simulink model "chaser_target_slosh"  (R2024a)
settings: Solver=VariableStepAuto  StartTime=0.0  StopTime=10.0  RelTol=1e-3
values from neighbouring files (symbols this model uses):
  dispslosh = 0.2    [main.m]
undefined symbols (not defined in the file or in its folder): chaser, InvDyn, KIN, reaction_wheels, slosh, solar_panel_big_reduced_FEM, solar_panel_target_reduced_FEM, target, ureal, uss, wn_big, wn_target
libraries: RCTblocks x54, SDTlibV1 x44
(part 2 of 3)

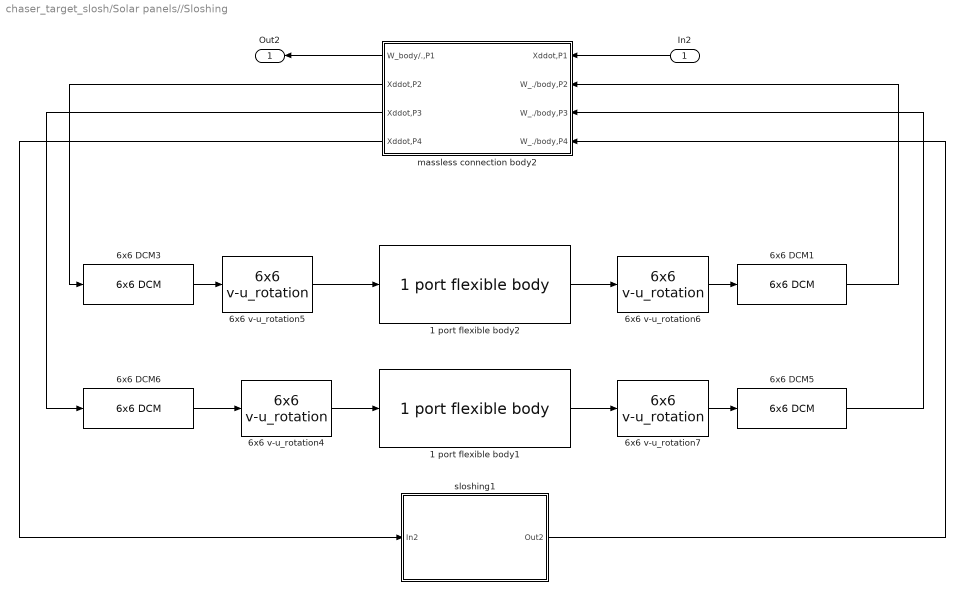
== system chaser_target_slosh/Solar panels//Sloshing ==
  In2 : Inport
  1 port flexible body1 : SDTlibV1/6 dof bodies/1 port flexible body  m=solar_panel_big_reduced_FEM.m  Ig=inertias_big  OG=r_PG_big  OP=[0;0;0]  n=6  xi=solar_panel_big_reduced_FEM.xi  w1=ureal('wnbig1',wn_big(1),'Percentage',20);  L11=solar_panel_big_reduced_FEM.L(1,1)  L12=solar_panel_big_reduced_FEM.L(1,2)  L13=solar_panel_big_reduced_FEM.L(1,3)  L14=solar_panel_big_reduced_FEM.L(1,4)  L15=solar_panel_big_reduced_FEM.L(1,5)  L16=solar_panel_big_reduced_FEM.L(1,6)  w2=wn_big(2)  L21=solar_panel_big_reduced_FEM.L(2,1)  L22=solar_panel_big_reduced_FEM.L(2,2)  L23=solar_panel_big_reduced_FEM.L(2,3)  L24=solar_panel_big_reduced_FEM.L(2,4)  L25=solar_panel_big_reduced_FEM.L(2,5)  L26=solar_panel_big_reduced_FEM.L(2,6)  w3=wn_big(3)  L31=solar_panel_big_reduced_FEM.L(3,1)  L32=solar_panel_big_reduced_FEM.L(3,2)  L33=solar_panel_big_reduced_FEM.L(3,3)  L34=solar_panel_big_reduced_FEM.L(3,4)  L35=solar_panel_big_reduced_FEM.L(3,5)  L36=solar_panel_big_reduced_FEM.L(3,6)  w4=wn_big(4)  L41=solar_panel_big_reduced_FEM.L(4,1)  L42=solar_panel_big_reduced_FEM.L(4,2)  L43=solar_panel_big_reduced_FEM.L(4,3)  L44=solar_panel_big_reduced_FEM.L(4,4)  L45=solar_panel_big_reduced_FEM.L(4,5)  L46=solar_panel_big_reduced_FEM.L(4,6)  w5=wn_big(5)  L51=solar_panel_big_reduced_FEM.L(5,1)  L52=solar_panel_big_reduced_FEM.L(5,2)  L53=solar_panel_big_reduced_FEM.L(5,3)  L54=solar_panel_big_reduced_FEM.L(5,4)  L55=solar_panel_big_reduced_FEM.L(5,5)  L56=solar_panel_big_reduced_FEM.L(5,6)  w6=wn_big(6)  L61=solar_panel_big_reduced_FEM.L(6,1)  L62=solar_panel_big_reduced_FEM.L(6,2)  L63=solar_panel_big_reduced_FEM.L(6,3)  L64=solar_panel_big_reduced_FEM.L(6,4)  L65=solar_panel_big_reduced_FEM.L(6,5)  L66=solar_panel_big_reduced_FEM.L(6,6)  w7=0  L71=0  L72=0  L73=0  L74=0  L75=0  L76=0  w8=0  L81=0  L82=0  L83=0  L84=0  L85=0  L86=0  w9=0  L91=0  L92=0  L93=0  L94=0  L95=0  L96=0  w10=0  L101=0  L102=0  L103=0  L104=0  L105=0  L106=0
      settings: SourceProductName=SDTlib
  1 port flexible body2 : SDTlibV1/6 dof bodies/1 port flexible body  m=solar_panel_big_reduced_FEM.m  Ig=inertias_big  OG=r_PG_big  OP=[0;0;0]  n=6  xi=solar_panel_big_reduced_FEM.xi  w1=ureal('wnbig1',wn_big(1),'Percentage',20);  L11=solar_panel_big_reduced_FEM.L(1,1)  L12=solar_panel_big_reduced_FEM.L(1,2)  L13=solar_panel_big_reduced_FEM.L(1,3)  L14=solar_panel_big_reduced_FEM.L(1,4)  L15=solar_panel_big_reduced_FEM.L(1,5)  L16=solar_panel_big_reduced_FEM.L(1,6)  w2=wn_big(2)  L21=solar_panel_big_reduced_FEM.L(2,1)  L22=solar_panel_big_reduced_FEM.L(2,2)  L23=solar_panel_big_reduced_FEM.L(2,3)  L24=solar_panel_big_reduced_FEM.L(2,4)  L25=solar_panel_big_reduced_FEM.L(2,5)  L26=solar_panel_big_reduced_FEM.L(2,6)  w3=wn_big(3)  L31=solar_panel_big_reduced_FEM.L(3,1)  L32=solar_panel_big_reduced_FEM.L(3,2)  L33=solar_panel_big_reduced_FEM.L(3,3)  L34=solar_panel_big_reduced_FEM.L(3,4)  L35=solar_panel_big_reduced_FEM.L(3,5)  L36=solar_panel_big_reduced_FEM.L(3,6)  w4=wn_big(4)  L41=solar_panel_big_reduced_FEM.L(4,1)  L42=solar_panel_big_reduced_FEM.L(4,2)  L43=solar_panel_big_reduced_FEM.L(4,3)  L44=solar_panel_big_reduced_FEM.L(4,4)  L45=solar_panel_big_reduced_FEM.L(4,5)  L46=solar_panel_big_reduced_FEM.L(4,6)  w5=wn_big(5)  L51=solar_panel_big_reduced_FEM.L(5,1)  L52=solar_panel_big_reduced_FEM.L(5,2)  L53=solar_panel_big_reduced_FEM.L(5,3)  L54=solar_panel_big_reduced_FEM.L(5,4)  L55=solar_panel_big_reduced_FEM.L(5,5)  L56=solar_panel_big_reduced_FEM.L(5,6)  w6=wn_big(6)  L61=solar_panel_big_reduced_FEM.L(6,1)  L62=solar_panel_big_reduced_FEM.L(6,2)  L63=solar_panel_big_reduced_FEM.L(6,3)  L64=solar_panel_big_reduced_FEM.L(6,4)  L65=solar_panel_big_reduced_FEM.L(6,5)  L66=solar_panel_big_reduced_FEM.L(6,6)  w7=0  L71=0  L72=0  L73=0  L74=0  L75=0  L76=0  w8=0  L81=0  L82=0  L83=0  L84=0  L85=0  L86=0  w9=0  L91=0  L92=0  L93=0  L94=0  L95=0  L96=0  w10=0  L101=0  L102=0  L103=0  L104=0  L105=0  L106=0
      settings: SourceProductName=SDTlib
  6x6 DCM1 : SDTlibV1/3//6 dof DCM/6x6 DCM  rot=chaser.solarpanel.R(:,:,1)  transp=off
      settings: SourceProductName=SDTlib
  6x6 DCM3 : SDTlibV1/3//6 dof DCM/6x6 DCM  rot=chaser.solarpanel.R(:,:,1)  transp=on
      settings: SourceProductName=SDTlib
  6x6 DCM5 : SDTlibV1/3//6 dof DCM/6x6 DCM  rot=chaser.solarpanel.R(:,:,2)  transp=off
      settings: SourceProductName=SDTlib
  6x6 DCM6 : SDTlibV1/3//6 dof DCM/6x6 DCM  rot=chaser.solarpanel.R(:,:,2)  transp=on
      settings: SourceProductName=SDTlib
  6x6 v-u_rotation4 : SDTlibV1/3//6 dof DCM/6x6 v-u_rotation  ra=[0;1;0]  theta=ureal('theta8',0,'Range',[-pi pi])  transp=on
      settings: SourceProductName=SDTlib
  6x6 v-u_rotation5 : SDTlibV1/3//6 dof DCM/6x6 v-u_rotation  ra=[0;1;0]  theta=ureal('theta7',0,'Range',[-pi pi])  transp=on
      settings: SourceProductName=SDTlib
  6x6 v-u_rotation6 : SDTlibV1/3//6 dof DCM/6x6 v-u_rotation  ra=[0;1;0]  theta=ureal('theta7',0,'Range',[-pi pi])  transp=off
      settings: SourceProductName=SDTlib
  6x6 v-u_rotation7 : SDTlibV1/3//6 dof DCM/6x6 v-u_rotation  ra=[0;1;0]  theta=ureal('theta8',0,'Range',[-pi pi])  transp=off
      settings: SourceProductName=SDTlib
  massless connection body2 : Subsystem  mask(Massless multi_port (6nx6n)){n=4, numinv=1, OP1=[0;0;0], OP2=chaser.solarpanel.location(:,1)*0.9, OP3=chaser.solarpanel.location(:,2)*0.9, OP4=[0;0;0], OP5=chaser.GNC.control.reaction_wheels.positions(:,4), OP6=[0;0;0], OP7=[0;0;0]}
      mask prompts: n "Number of ports"; numinv "Port (point) Pj: j="; OP1 "OP1 (3x1 vector, m)"; OP2 "OP2 (3x1 vector, m)"; OP3 "OP3 (3x1 vector, m)"; OP4 "OP4 (3x1 vector, m)"; OP5 "OP5 (3x1 vector,m)"; OP6 "OP6 (3x1 vector,m)"; OP7 "OP7 (3x1 vector,m)"
      mask help:
      | Massless body to transport wrenches and acceleration twists:
      | 6nx6n gain from:
      |  * the acceleration twist at one point Pj; i.e. the parent port,
      |  * the wrenches applied to this massless body at the n-1 points Pi (i=1,..n, except j); i.e. the child ports
      | to:
      |  * the wrench applied at point Pj by this massless body,
      |  * the accelaretion twists at the other n-1  points Pi (i=1,..n, except j).
      |
      | 0: the reference point
      | Pi (i=1:n): the n given connection points or ports (1<n<8).
      |
      | All parameters are expressed in the body frame.
      | Each parameter can be an uncertain parameter declared with "ureal"
      mask init:
      | MasslessConnectionBody
      mask Help: web('DocMassLessBody.html')
      mask TypeOptions n: 2 | 3 | 4 | 5 | 6 | 7
      mask TypeOptions numinv: 1 | 2 | 3 | 4 | 5 | 6 | 7
      mask DialogControl ParameterGroupVar Prompt: Main parameters
      mask DialogControl port1 Prompt: Port #1
      mask DialogControl port2 Prompt: #2
      mask DialogControl port3 Prompt: #3
      mask DialogControl port4 Prompt: #4
      mask DialogControl port5 Prompt: #5
      mask DialogControl port6 Prompt: #6
      mask DialogControl port7 Prompt: #7
      mask Display:
      | disp('Massless\n connection body\n (6nx6n)')
      | for ii=1:n+1
      |     if numinv==ii,
      |         port_label('output',ii,['W_body/.,P',num2str(ii)])
      |         port_label('input', ii,['Xddot,P',num2str(ii)])
      |     else
      |         port_label('input', ii,['W_./body,P',num2str(ii)])
      |         port_label('output',ii,['Xddot,P',num2str(ii)])
      |     end
      | end
  sloshing1 : Subsystem
  Out2 : Outport
  wires:
  massless connection body2/1(W_body/.,P1) -> Out2/1
  In2/1 -> massless connection body2/1(Xddot,P1)
  1 port flexible body2/1 -> 6x6 v-u_rotation6/1
  6x6 v-u_rotation5/1 -> 1 port flexible body2/1
  6x6 v-u_rotation6/1 -> 6x6 DCM1/1
  1 port flexible body1/1 -> 6x6 v-u_rotation7/1
  massless connection body2/2(Xddot,P2) -> 6x6 DCM3/1
  6x6 DCM1/1 -> massless connection body2/2(W_./body,P2)
  6x6 DCM3/1 -> 6x6 v-u_rotation5/1
  6x6 v-u_rotation7/1 -> 6x6 DCM5/1
  6x6 DCM5/1 -> massless connection body2/3(W_./body,P3)
  massless connection body2/3(Xddot,P3) -> 6x6 DCM6/1
  6x6 DCM6/1 -> 6x6 v-u_rotation4/1
  6x6 v-u_rotation4/1 -> 1 port flexible body1/1
  massless connection body2/4(Xddot,P4) -> sloshing1/1(In2)
  sloshing1/1(Out2) -> massless connection body2/4(W_./body,P4)

== system chaser_target_slosh/Reaction Wheels 0 vel1/RW1 ==
  Xddot : Inport  PortDimensions=6
  Demux : Demux  Outputs=[3 3]
  Gain1 : Gain  Gain=pass'  Multiplication=Matrix(K*u) (u vector)
  Gain2 : Gain  Gain=pass  Multiplication=Matrix(K*u) (u vector)
  Gain3 : Gain  Gain=m*eye(3)  Multiplication=Matrix(K*u) (u vector)
  Gain4 : Gain  Gain=diag([Ir Ir Iw])  Multiplication=Matrix(K*u) (u vector)
  Gain8 : Gain  Gain=-Tau_GP'  Multiplication=Matrix(K*u) (u vector)
  Gain9 : Gain  Gain=Tau_GP  Multiplication=Matrix(K*u) (u vector)
  Mux : Mux  Inputs=[3 3]
  W_body/. : Outport  VectorParamsAs1DForOutWhenUnconnected=off
  wires:
  Gain3/1 -> Mux/1
  Gain2/1 -> Mux/2
  Demux/1 -> Gain3/1
  Demux/2 -> Gain1/1
  Gain1/1 -> Gain4/1
  Gain4/1 -> Gain2/1
  Gain8/1 -> W_body/./1
  Mux/1 -> Gain8/1
  Gain9/1 -> Demux/1
  Xddot/1 -> Gain9/1

== system chaser_target_slosh/Reaction Wheels 0 vel1/RW2 ==
  Xddot : Inport  PortDimensions=6
  Demux : Demux  Outputs=[3 3]
  Gain1 : Gain  Gain=pass'  Multiplication=Matrix(K*u) (u vector)
  Gain2 : Gain  Gain=pass  Multiplication=Matrix(K*u) (u vector)
  Gain3 : Gain  Gain=m*eye(3)  Multiplication=Matrix(K*u) (u vector)
  Gain4 : Gain  Gain=diag([Ir Ir Iw])  Multiplication=Matrix(K*u) (u vector)
  Gain8 : Gain  Gain=-Tau_GP'  Multiplication=Matrix(K*u) (u vector)
  Gain9 : Gain  Gain=Tau_GP  Multiplication=Matrix(K*u) (u vector)
  Mux : Mux  Inputs=[3 3]
  W_body/. : Outport  VectorParamsAs1DForOutWhenUnconnected=off
  wires:
  Gain3/1 -> Mux/1
  Gain2/1 -> Mux/2
  Demux/1 -> Gain3/1
  Demux/2 -> Gain1/1
  Gain1/1 -> Gain4/1
  Gain4/1 -> Gain2/1
  Gain8/1 -> W_body/./1
  Mux/1 -> Gain8/1
  Gain9/1 -> Demux/1
  Xddot/1 -> Gain9/1

== system chaser_target_slosh/Reaction Wheels 0 vel1/RW3 ==
  Xddot : Inport  PortDimensions=6
  Demux : Demux  Outputs=[3 3]
  Gain1 : Gain  Gain=pass'  Multiplication=Matrix(K*u) (u vector)
  Gain2 : Gain  Gain=pass  Multiplication=Matrix(K*u) (u vector)
  Gain3 : Gain  Gain=m*eye(3)  Multiplication=Matrix(K*u) (u vector)
  Gain4 : Gain  Gain=diag([Ir Ir Iw])  Multiplication=Matrix(K*u) (u vector)
  Gain8 : Gain  Gain=-Tau_GP'  Multiplication=Matrix(K*u) (u vector)
  Gain9 : Gain  Gain=Tau_GP  Multiplication=Matrix(K*u) (u vector)
  Mux : Mux  Inputs=[3 3]
  W_body/. : Outport  VectorParamsAs1DForOutWhenUnconnected=off
  wires:
  Gain3/1 -> Mux/1
  Gain2/1 -> Mux/2
  Demux/1 -> Gain3/1
  Demux/2 -> Gain1/1
  Gain1/1 -> Gain4/1
  Gain4/1 -> Gain2/1
  Gain8/1 -> W_body/./1
  Mux/1 -> Gain8/1
  Gain9/1 -> Demux/1
  Xddot/1 -> Gain9/1

== system chaser_target_slosh/Reaction Wheels 0 vel1/RW4 ==
  Xddot : Inport  PortDimensions=6
  Demux : Demux  Outputs=[3 3]
  Gain1 : Gain  Gain=pass'  Multiplication=Matrix(K*u) (u vector)
  Gain2 : Gain  Gain=pass  Multiplication=Matrix(K*u) (u vector)
  Gain3 : Gain  Gain=m*eye(3)  Multiplication=Matrix(K*u) (u vector)
  Gain4 : Gain  Gain=diag([Ir Ir Iw])  Multiplication=Matrix(K*u) (u vector)
  Gain8 : Gain  Gain=-Tau_GP'  Multiplication=Matrix(K*u) (u vector)
  Gain9 : Gain  Gain=Tau_GP  Multiplication=Matrix(K*u) (u vector)
  Mux : Mux  Inputs=[3 3]
  W_body/. : Outport  VectorParamsAs1DForOutWhenUnconnected=off
  wires:
  Gain3/1 -> Mux/1
  Gain2/1 -> Mux/2
  Demux/1 -> Gain3/1
  Demux/2 -> Gain1/1
  Gain1/1 -> Gain4/1
  Gain4/1 -> Gain2/1
  Gain8/1 -> W_body/./1
  Mux/1 -> Gain8/1
  Gain9/1 -> Demux/1
  Xddot/1 -> Gain9/1

== system chaser_target_slosh/Reaction Wheels 0 vel1/massless connection body1 ==
  Xddot,P1 : Inport  PortDimensions=6
  W_./body,P2 : Inport  Port=2  PortDimensions=6
  W_./body,P3 : Inport  Port=3  PortDimensions=6
  W_./body,P4 : Inport  Port=4  PortDimensions=6
  W_./body,P5 : Inport  Port=5  PortDimensions=6
  Demux : Demux  Outputs=[6 6 6 6 6]
  Gain : RCTblocks/Uncertain State Space  Tag=USS  USystem=uss(KIN)  UValue=[]  X0=[]  uX0=[]
  Mux : Mux  Inputs=[6 6 6 6 6]
  W_body/.,P1 : Outport
  Xddot,P2 : Outport  Port=2
  Xddot,P3 : Outport  Port=3
  Xddot,P4 : Outport  Port=4
  Xddot,P5 : Outport  Port=5
  wires:
  Mux/1 -> Gain/1
  Gain/1 -> Demux/1
  Xddot,P1/1 -> Mux/1
  Demux/1 -> W_body/.,P1/1
  W_./body,P2/1 -> Mux/2
  Demux/2 -> Xddot,P2/1
  W_./body,P3/1 -> Mux/3
  Demux/3 -> Xddot,P3/1
  W_./body,P4/1 -> Mux/4
  Demux/4 -> Xddot,P4/1
  W_./body,P5/1 -> Mux/5
  Demux/5 -> Xddot,P5/1

== system chaser_target_slosh/Robotic arm/Multi port rigid body1 ==
  Xddot,P1 : Inport  PortDimensions=6
  W_./body,P2 : Inport  Port=2  PortDimensions=6
  Demux : Demux  Outputs=[6 6]
  Gain : RCTblocks/Uncertain State Space  Tag=USS  USystem=uss(InvDyn)  UValue=[]  X0=[]  uX0=[]
  Mux : Mux  Inputs=[6 6]
  W_body/.,P1 : Outport
  Xddot,P2 : Outport  Port=2
  wires:
  Mux/1 -> Gain/1
  Gain/1 -> Demux/1
  Xddot,P1/1 -> Mux/1
  Demux/1 -> W_body/.,P1/1
  W_./body,P2/1 -> Mux/2
  Demux/2 -> Xddot,P2/1

== system chaser_target_slosh/Robotic arm/Multi port rigid body3 ==
  Xddot,P1 : Inport  PortDimensions=6
  W_./body,P2 : Inport  Port=2  PortDimensions=6
  Demux : Demux  Outputs=[6 6]
  Gain : RCTblocks/Uncertain State Space  Tag=USS  USystem=uss(InvDyn)  UValue=[]  X0=[]  uX0=[]
  Mux : Mux  Inputs=[6 6]
  W_body/.,P1 : Outport
  Xddot,P2 : Outport  Port=2
  wires:
  Mux/1 -> Gain/1
  Gain/1 -> Demux/1
  Xddot,P1/1 -> Mux/1
  Demux/1 -> W_body/.,P1/1
  W_./body,P2/1 -> Mux/2
  Demux/2 -> Xddot,P2/1

== system chaser_target_slosh/Robotic arm/Multi port rigid body4 ==
  Xddot,P1 : Inport  PortDimensions=6
  W_./body,P2 : Inport  Port=2  PortDimensions=6
  Demux : Demux  Outputs=[6 6]
  Gain : RCTblocks/Uncertain State Space  Tag=USS  USystem=uss(InvDyn)  UValue=[]  X0=[]  uX0=[]
  Mux : Mux  Inputs=[6 6]
  W_body/.,P1 : Outport
  Xddot,P2 : Outport  Port=2
  wires:
  Mux/1 -> Gain/1
  Gain/1 -> Demux/1
  Xddot,P1/1 -> Mux/1
  Demux/1 -> W_body/.,P1/1
  W_./body,P2/1 -> Mux/2
  Demux/2 -> Xddot,P2/1

== system chaser_target_slosh/Robotic arm/Multi port rigid body6 ==
  Xddot,P1 : Inport  PortDimensions=6
  W_./body,P2 : Inport  Port=2  PortDimensions=6
  Demux : Demux  Outputs=[6 6]
  Gain : RCTblocks/Uncertain State Space  Tag=USS  USystem=uss(InvDyn)  UValue=[]  X0=[]  uX0=[]
  Mux : Mux  Inputs=[6 6]
  W_body/.,P1 : Outport
  Xddot,P2 : Outport  Port=2
  wires:
  Mux/1 -> Gain/1
  Gain/1 -> Demux/1
  Xddot,P1/1 -> Mux/1
  Demux/1 -> W_body/.,P1/1
  W_./body,P2/1 -> Mux/2
  Demux/2 -> Xddot,P2/1

== system chaser_target_slosh/Robotic arm/Multi port rigid body7 ==
  Xddot,P1 : Inport  PortDimensions=6
  W_./body,P2 : Inport  Port=2  PortDimensions=6
  Demux : Demux  Outputs=[6 6]
  Gain : RCTblocks/Uncertain State Space  Tag=USS  USystem=uss(InvDyn)  UValue=[]  X0=[]  uX0=[]
  Mux : Mux  Inputs=[6 6]
  W_body/.,P1 : Outport
  Xddot,P2 : Outport  Port=2
  wires:
  Mux/1 -> Gain/1
  Gain/1 -> Demux/1
  Xddot,P1/1 -> Mux/1
  Demux/1 -> W_body/.,P1/1
  W_./body,P2/1 -> Mux/2
  Demux/2 -> Xddot,P2/1

== system chaser_target_slosh/Robotic arm/Multi port rigid body8 ==
  Xddot,P1 : Inport  PortDimensions=6
  W_./body,P2 : Inport  Port=2  PortDimensions=6
  Demux : Demux  Outputs=[6 6]
  Gain : RCTblocks/Uncertain State Space  Tag=USS  USystem=uss(InvDyn)  UValue=[]  X0=[]  uX0=[]
  Mux : Mux  Inputs=[6 6]
  W_body/.,P1 : Outport
  Xddot,P2 : Outport  Port=2
  wires:
  Mux/1 -> Gain/1
  Gain/1 -> Demux/1
  Xddot,P1/1 -> Mux/1
  Demux/1 -> W_body/.,P1/1
  W_./body,P2/1 -> Mux/2
  Demux/2 -> Xddot,P2/1

== system chaser_target_slosh/Robotic arm/Multi port rigid body9 ==
  Xddot,P1 : Inport  PortDimensions=6
  W_./body,P2 : Inport  Port=2  PortDimensions=6
  Demux : Demux  Outputs=[6 6]
  Gain : RCTblocks/Uncertain State Space  Tag=USS  USystem=uss(InvDyn)  UValue=[]  X0=[]  uX0=[]
  Mux : Mux  Inputs=[6 6]
  W_body/.,P1 : Outport
  Xddot,P2 : Outport  Port=2
  wires:
  Mux/1 -> Gain/1
  Gain/1 -> Demux/1
  Xddot,P1/1 -> Mux/1
  Demux/1 -> W_body/.,P1/1
  W_./body,P2/1 -> Mux/2
  Demux/2 -> Xddot,P2/1

== system chaser_target_slosh/Solar panels target 1st/massless connection body2 ==
  Xddot,P1 : Inport  PortDimensions=6
  W_./body,P2 : Inport  Port=2  PortDimensions=6
  W_./body,P3 : Inport  Port=3  PortDimensions=6
  W_./body,P4 : Inport  Port=4  PortDimensions=6
  Demux : Demux  Outputs=[6 6 6 6]
  Gain : RCTblocks/Uncertain State Space  Tag=USS  USystem=uss(KIN)  UValue=[]  X0=[]  uX0=[]
  Mux : Mux  Inputs=[6 6 6 6]
  W_body/.,P1 : Outport
  Xddot,P2 : Outport  Port=2
  Xddot,P3 : Outport  Port=3
  Xddot,P4 : Outport  Port=4
  wires:
  Mux/1 -> Gain/1
  Gain/1 -> Demux/1
  Xddot,P1/1 -> Mux/1
  Demux/1 -> W_body/.,P1/1
  W_./body,P2/1 -> Mux/2
  Demux/2 -> Xddot,P2/1
  W_./body,P3/1 -> Mux/3
  Demux/3 -> Xddot,P3/1
  W_./body,P4/1 -> Mux/4
  Demux/4 -> Xddot,P4/1

== system chaser_target_slosh/Solar panels target 1st/sloshing1 ==
  In2 : Inport
  massless connection body1 : Subsystem  mask(Massless multi_port (6nx6n)){n=7, numinv=1, OP1=[0;0;0], OP2=[0;0;dispslosh], OP3=[0;0;-dispslosh], OP4=[0;dispslosh;0], OP5=[0;-dispslosh;0], OP6=[dispslosh;0;0], OP7=[-dispslosh;0;0]}
      mask prompts: n "Number of ports"; numinv "Port (point) Pj: j="; OP1 "OP1 (3x1 vector, m)"; OP2 "OP2 (3x1 vector, m)"; OP3 "OP3 (3x1 vector, m)"; OP4 "OP4 (3x1 vector, m)"; OP5 "OP5 (3x1 vector,m)"; OP6 "OP6 (3x1 vector,m)"; OP7 "OP7 (3x1 vector,m)"
      mask help:
      | Massless body to transport wrenches and acceleration twists:
      | 6nx6n gain from:
      |  * the acceleration twist at one point Pj; i.e. the parent port,
      |  * the wrenches applied to this massless body at the n-1 points Pi (i=1,..n, except j); i.e. the child ports
      | to:
      |  * the wrench applied at point Pj by this massless body,
      |  * the accelaretion twists at the other n-1  points Pi (i=1,..n, except j).
      |
      | 0: the reference point
      | Pi (i=1:n): the n given connection points or ports (1<n<8).
      |
      | All parameters are expressed in the body frame.
      | Each parameter can be an uncertain parameter declared with "ureal"
      mask init:
      | MasslessConnectionBody
      mask Help: web('DocMassLessBody.html')
      mask TypeOptions n: 2 | 3 | 4 | 5 | 6 | 7
      mask TypeOptions numinv: 1 | 2 | 3 | 4 | 5 | 6 | 7
      mask DialogControl ParameterGroupVar Prompt: Main parameters
      mask DialogControl port1 Prompt: Port #1
      mask DialogControl port2 Prompt: #2
      mask DialogControl port3 Prompt: #3
      mask DialogControl port4 Prompt: #4
      mask DialogControl port5 Prompt: #5
      mask DialogControl port6 Prompt: #6
      mask DialogControl port7 Prompt: #7
      mask Display:
      | disp('Massless\n connection body\n (6nx6n)')
      | for ii=1:n+1
      |     if numinv==ii,
      |         port_label('output',ii,['W_body/.,P',num2str(ii)])
      |         port_label('input', ii,['Xddot,P',num2str(ii)])
      |     else
      |         port_label('input', ii,['W_./body,P',num2str(ii)])
      |         port_label('output',ii,['Xddot,P',num2str(ii)])
      |     end
      | end
  zaxis1 : Subsystem  AncestorBlock=SDTlibV1/6 dof bodies/u_sloshing  mask(Sloshing 1D mass-spring model(6x6)){xi=slosh.cj_target, w1=slosh.kj_target, m1=slosh.mj_target3}
      mask prompts: xi "Damping ratio"; w1 "Frequency (rd/s)"; m1 "Sloshing mass attached to the spring  (kg)"
      mask help:
      | Simplified dynamic model of lateral sloshing with a spring-mass model located at point P (connection point with the hub):
      | 6x6 transfer between acceleretion twist at P and wrench applied by the spring-mass system at P. The model is expressed in the (inherit) body frame.
      |
      | v: the direction vector of the spring-mass system.
      | Each parameter (except v) can be an uncertain parameter declared with "ureal"
      mask init:
      | % pass=ra2DCMi(v)
      mask Help: web('Docsloshing.html')
      mask DialogControl ParameterGroupVar Prompt: Main parameters
      mask DialogControl damping Prompt: Damping ratio
      mask DialogControl mode1 Prompt: Flexible mode:
      mask Display:
      | disp('Sloshing 1D \n mass-spring \n model(6x6)')
      | port_label('input', 1, 'Xddot')
      | port_label('output', 1, 'W_body/.')
  zaxis2 : Subsystem  AncestorBlock=SDTlibV1/6 dof bodies/u_sloshing  mask(Sloshing 1D mass-spring model(6x6)){xi=slosh.cj_target, w1=slosh.kj_target, m1=slosh.mj_target4}
      mask prompts: xi "Damping ratio"; w1 "Frequency (rd/s)"; m1 "Sloshing mass attached to the spring  (kg)"
      mask help:
      | Simplified dynamic model of lateral sloshing with a spring-mass model located at point P (connection point with the hub):
      | 6x6 transfer between acceleretion twist at P and wrench applied by the spring-mass system at P. The model is expressed in the (inherit) body frame.
      |
      | v: the direction vector of the spring-mass system.
      | Each parameter (except v) can be an uncertain parameter declared with "ureal"
      mask init:
      | % pass=ra2DCMi(v)
      mask Help: web('Docsloshing.html')
      mask DialogControl ParameterGroupVar Prompt: Main parameters
      mask DialogControl damping Prompt: Damping ratio
      mask DialogControl mode1 Prompt: Flexible mode:
      mask Display:
      | disp('Sloshing 1D \n mass-spring \n model(6x6)')
      | port_label('input', 1, 'Xddot')
      | port_label('output', 1, 'W_body/.')
  zaxis3 : Subsystem  AncestorBlock=SDTlibV1/6 dof bodies/u_sloshing  mask(Sloshing 1D mass-spring model(6x6)){xi=slosh.cj_target, w1=slosh.kj_target, m1=slosh.mj_target5}
      mask prompts: xi "Damping ratio"; w1 "Frequency (rd/s)"; m1 "Sloshing mass attached to the spring  (kg)"
      mask help:
      | Simplified dynamic model of lateral sloshing with a spring-mass model located at point P (connection point with the hub):
      | 6x6 transfer between acceleretion twist at P and wrench applied by the spring-mass system at P. The model is expressed in the (inherit) body frame.
      |
      | v: the direction vector of the spring-mass system.
      | Each parameter (except v) can be an uncertain parameter declared with "ureal"
      mask init:
      | % pass=ra2DCMi(v)
      mask Help: web('Docsloshing.html')
      mask DialogControl ParameterGroupVar Prompt: Main parameters
      mask DialogControl damping Prompt: Damping ratio
      mask DialogControl mode1 Prompt: Flexible mode:
      mask Display:
      | disp('Sloshing 1D \n mass-spring \n model(6x6)')
      | port_label('input', 1, 'Xddot')
      | port_label('output', 1, 'W_body/.')
  zaxis4 : Subsystem  AncestorBlock=SDTlibV1/6 dof bodies/u_sloshing  mask(Sloshing 1D mass-spring model(6x6)){xi=slosh.cj_target, w1=slosh.kj_target, m1=slosh.mj_target6}
      mask prompts: xi "Damping ratio"; w1 "Frequency (rd/s)"; m1 "Sloshing mass attached to the spring  (kg)"
      mask help:
      | Simplified dynamic model of lateral sloshing with a spring-mass model located at point P (connection point with the hub):
      | 6x6 transfer between acceleretion twist at P and wrench applied by the spring-mass system at P. The model is expressed in the (inherit) body frame.
      |
      | v: the direction vector of the spring-mass system.
      | Each parameter (except v) can be an uncertain parameter declared with "ureal"
      mask init:
      | % pass=ra2DCMi(v)
      mask Help: web('Docsloshing.html')
      mask DialogControl ParameterGroupVar Prompt: Main parameters
      mask DialogControl damping Prompt: Damping ratio
      mask DialogControl mode1 Prompt: Flexible mode:
      mask Display:
      | disp('Sloshing 1D \n mass-spring \n model(6x6)')
      | port_label('input', 1, 'Xddot')
      | port_label('output', 1, 'W_body/.')
  zaxis5 : Subsystem  AncestorBlock=SDTlibV1/6 dof bodies/u_sloshing  mask(Sloshing 1D mass-spring model(6x6)){xi=slosh.cj_target, w1=slosh.kj_target, m1=slosh.mj_target2}
      mask prompts: xi "Damping ratio"; w1 "Frequency (rd/s)"; m1 "Sloshing mass attached to the spring  (kg)"
      mask help:
      | Simplified dynamic model of lateral sloshing with a spring-mass model located at point P (connection point with the hub):
      | 6x6 transfer between acceleretion twist at P and wrench applied by the spring-mass system at P. The model is expressed in the (inherit) body frame.
      |
      | v: the direction vector of the spring-mass system.
      | Each parameter (except v) can be an uncertain parameter declared with "ureal"
      mask init:
      | % pass=ra2DCMi(v)
      mask Help: web('Docsloshing.html')
      mask DialogControl ParameterGroupVar Prompt: Main parameters
      mask DialogControl damping Prompt: Damping ratio
      mask DialogControl mode1 Prompt: Flexible mode:
      mask Display:
      | disp('Sloshing 1D \n mass-spring \n model(6x6)')
      | port_label('input', 1, 'Xddot')
      | port_label('output', 1, 'W_body/.')
  zaxis6 : Subsystem  AncestorBlock=SDTlibV1/6 dof bodies/u_sloshing  mask(Sloshing 1D mass-spring model(6x6)){xi=slosh.cj_target, w1=slosh.kj_target, m1=slosh.mj_target}
      mask prompts: xi "Damping ratio"; w1 "Frequency (rd/s)"; m1 "Sloshing mass attached to the spring  (kg)"
      mask help:
      | Simplified dynamic model of lateral sloshing with a spring-mass model located at point P (connection point with the hub):
      | 6x6 transfer between acceleretion twist at P and wrench applied by the spring-mass system at P. The model is expressed in the (inherit) body frame.
      |
      | v: the direction vector of the spring-mass system.
      | Each parameter (except v) can be an uncertain parameter declared with "ureal"
      mask init:
      | % pass=ra2DCMi(v)
      mask Help: web('Docsloshing.html')
      mask DialogControl ParameterGroupVar Prompt: Main parameters
      mask DialogControl damping Prompt: Damping ratio
      mask DialogControl mode1 Prompt: Flexible mode:
      mask Display:
      | disp('Sloshing 1D \n mass-spring \n model(6x6)')
      | port_label('input', 1, 'Xddot')
      | port_label('output', 1, 'W_body/.')
  Out2 : Outport
  wires:
  massless connection body1/1(W_body/.,P1) -> Out2/1
  In2/1 -> massless connection body1/1(Xddot,P1)
  massless connection body1/2(Xddot,P2) -> zaxis6/1(Xddot)
  zaxis6/1(W_body/.) -> massless connection body1/2(W_./body,P2)
  massless connection body1/3(Xddot,P3) -> zaxis5/1(Xddot)
  zaxis5/1(W_body/.) -> massless connection body1/3(W_./body,P3)
  zaxis1/1(W_body/.) -> massless connection body1/4(W_./body,P4)
  zaxis2/1(W_body/.) -> massless connection body1/5(W_./body,P5)
  zaxis3/1(W_body/.) -> massless connection body1/6(W_./body,P6)
  zaxis4/1(W_body/.) -> massless connection body1/7(W_./body,P7)
  massless connection body1/4(Xddot,P4) -> zaxis1/1(Xddot)
  massless connection body1/5(Xddot,P5) -> zaxis2/1(Xddot)
  massless connection body1/6(Xddot,P6) -> zaxis3/1(Xddot)
  massless connection body1/7(Xddot,P7) -> zaxis4/1(Xddot)

== system chaser_target_slosh/Solar panels//Sloshing/massless connection body2 ==
  Xddot,P1 : Inport  PortDimensions=6
  W_./body,P2 : Inport  Port=2  PortDimensions=6
  W_./body,P3 : Inport  Port=3  PortDimensions=6
  W_./body,P4 : Inport  Port=4  PortDimensions=6
  Demux : Demux  Outputs=[6 6 6 6]
  Gain : RCTblocks/Uncertain State Space  Tag=USS  USystem=uss(KIN)  UValue=[]  X0=[]  uX0=[]
  Mux : Mux  Inputs=[6 6 6 6]
  W_body/.,P1 : Outport
  Xddot,P2 : Outport  Port=2
  Xddot,P3 : Outport  Port=3
  Xddot,P4 : Outport  Port=4
  wires:
  Mux/1 -> Gain/1
  Gain/1 -> Demux/1
  Xddot,P1/1 -> Mux/1
  Demux/1 -> W_body/.,P1/1
  W_./body,P2/1 -> Mux/2
  Demux/2 -> Xddot,P2/1
  W_./body,P3/1 -> Mux/3
  Demux/3 -> Xddot,P3/1
  W_./body,P4/1 -> Mux/4
  Demux/4 -> Xddot,P4/1

== system chaser_target_slosh/Solar panels//Sloshing/sloshing1 ==
  In2 : Inport
  massless connection body1 : Subsystem  mask(Massless multi_port (6nx6n)){n=7, numinv=1, OP1=[0;0;0], OP2=[0;0;dispslosh], OP3=[0;0;-dispslosh], OP4=[0;dispslosh;0], OP5=[0;-dispslosh;0], OP6=[dispslosh;0;0], OP7=[-dispslosh;0;0]}
      mask prompts: n "Number of ports"; numinv "Port (point) Pj: j="; OP1 "OP1 (3x1 vector, m)"; OP2 "OP2 (3x1 vector, m)"; OP3 "OP3 (3x1 vector, m)"; OP4 "OP4 (3x1 vector, m)"; OP5 "OP5 (3x1 vector,m)"; OP6 "OP6 (3x1 vector,m)"; OP7 "OP7 (3x1 vector,m)"
      mask help:
      | Massless body to transport wrenches and acceleration twists:
      | 6nx6n gain from:
      |  * the acceleration twist at one point Pj; i.e. the parent port,
      |  * the wrenches applied to this massless body at the n-1 points Pi (i=1,..n, except j); i.e. the child ports
      | to:
      |  * the wrench applied at point Pj by this massless body,
      |  * the accelaretion twists at the other n-1  points Pi (i=1,..n, except j).
      |
      | 0: the reference point
      | Pi (i=1:n): the n given connection points or ports (1<n<8).
      |
      | All parameters are expressed in the body frame.
      | Each parameter can be an uncertain parameter declared with "ureal"
      mask init:
      | MasslessConnectionBody
      mask Help: web('DocMassLessBody.html')
      mask TypeOptions n: 2 | 3 | 4 | 5 | 6 | 7
      mask TypeOptions numinv: 1 | 2 | 3 | 4 | 5 | 6 | 7
      mask DialogControl ParameterGroupVar Prompt: Main parameters
      mask DialogControl port1 Prompt: Port #1
      mask DialogControl port2 Prompt: #2
      mask DialogControl port3 Prompt: #3
      mask DialogControl port4 Prompt: #4
      mask DialogControl port5 Prompt: #5
      mask DialogControl port6 Prompt: #6
      mask DialogControl port7 Prompt: #7
      mask Display:
      | disp('Massless\n connection body\n (6nx6n)')
      | for ii=1:n+1
      |     if numinv==ii,
      |         port_label('output',ii,['W_body/.,P',num2str(ii)])
      |         port_label('input', ii,['Xddot,P',num2str(ii)])
      |     else
      |         port_label('input', ii,['W_./body,P',num2str(ii)])
      |         port_label('output',ii,['Xddot,P',num2str(ii)])
      |     end
      | end
  zaxis1 : Subsystem  AncestorBlock=SDTlibV1/6 dof bodies/u_sloshing  mask(Sloshing 1D mass-spring model(6x6)){xi=slosh.cj, w1=slosh.kj, m1=slosh.mj2}
      mask prompts: xi "Damping ratio"; w1 "Frequency (rd/s)"; m1 "Sloshing mass attached to the spring  (kg)"
      mask help:
      | Simplified dynamic model of lateral sloshing with a spring-mass model located at point P (connection point with the hub):
      | 6x6 transfer between acceleretion twist at P and wrench applied by the spring-mass system at P. The model is expressed in the (inherit) body frame.
      |
      | v: the direction vector of the spring-mass system.
      | Each parameter (except v) can be an uncertain parameter declared with "ureal"
      mask init:
      | % pass=ra2DCMi(v)
      mask Help: web('Docsloshing.html')
      mask DialogControl ParameterGroupVar Prompt: Main parameters
      mask DialogControl damping Prompt: Damping ratio
      mask DialogControl mode1 Prompt: Flexible mode:
      mask Display:
      | disp('Sloshing 1D \n mass-spring \n model(6x6)')
      | port_label('input', 1, 'Xddot')
      | port_label('output', 1, 'W_body/.')
  zaxis2 : Subsystem  AncestorBlock=SDTlibV1/6 dof bodies/u_sloshing  mask(Sloshing 1D mass-spring model(6x6)){xi=slosh.cj, w1=slosh.kj, m1=slosh.mj5}
      mask prompts: xi "Damping ratio"; w1 "Frequency (rd/s)"; m1 "Sloshing mass attached to the spring  (kg)"
      mask help:
      | Simplified dynamic model of lateral sloshing with a spring-mass model located at point P (connection point with the hub):
      | 6x6 transfer between acceleretion twist at P and wrench applied by the spring-mass system at P. The model is expressed in the (inherit) body frame.
      |
      | v: the direction vector of the spring-mass system.
      | Each parameter (except v) can be an uncertain parameter declared with "ureal"
      mask init:
      | % pass=ra2DCMi(v)
      mask Help: web('Docsloshing.html')
      mask DialogControl ParameterGroupVar Prompt: Main parameters
      mask DialogControl damping Prompt: Damping ratio
      mask DialogControl mode1 Prompt: Flexible mode:
      mask Display:
      | disp('Sloshing 1D \n mass-spring \n model(6x6)')
      | port_label('input', 1, 'Xddot')
      | port_label('output', 1, 'W_body/.')
  zaxis3 : Subsystem  AncestorBlock=SDTlibV1/6 dof bodies/u_sloshing  mask(Sloshing 1D mass-spring model(6x6)){xi=slosh.cj, w1=slosh.kj, m1=slosh.mj4}
      mask prompts: xi "Damping ratio"; w1 "Frequency (rd/s)"; m1 "Sloshing mass attached to the spring  (kg)"
      mask help:
      | Simplified dynamic model of lateral sloshing with a spring-mass model located at point P (connection point with the hub):
      | 6x6 transfer between acceleretion twist at P and wrench applied by the spring-mass system at P. The model is expressed in the (inherit) body frame.
      |
      | v: the direction vector of the spring-mass system.
      | Each parameter (except v) can be an uncertain parameter declared with "ureal"
      mask init:
      | % pass=ra2DCMi(v)
      mask Help: web('Docsloshing.html')
      mask DialogControl ParameterGroupVar Prompt: Main parameters
      mask DialogControl damping Prompt: Damping ratio
      mask DialogControl mode1 Prompt: Flexible mode:
      mask Display:
      | disp('Sloshing 1D \n mass-spring \n model(6x6)')
      | port_label('input', 1, 'Xddot')
      | port_label('output', 1, 'W_body/.')
  zaxis4 : Subsystem  AncestorBlock=SDTlibV1/6 dof bodies/u_sloshing  mask(Sloshing 1D mass-spring model(6x6)){xi=slosh.cj, w1=slosh.kj, m1=slosh.mj3}
      mask prompts: xi "Damping ratio"; w1 "Frequency (rd/s)"; m1 "Sloshing mass attached to the spring  (kg)"
      mask help:
      | Simplified dynamic model of lateral sloshing with a spring-mass model located at point P (connection point with the hub):
      | 6x6 transfer between acceleretion twist at P and wrench applied by the spring-mass system at P. The model is expressed in the (inherit) body frame.
      |
      | v: the direction vector of the spring-mass system.
      | Each parameter (except v) can be an uncertain parameter declared with "ureal"
      mask init:
      | % pass=ra2DCMi(v)
      mask Help: web('Docsloshing.html')
      mask DialogControl ParameterGroupVar Prompt: Main parameters
      mask DialogControl damping Prompt: Damping ratio
      mask DialogControl mode1 Prompt: Flexible mode:
      mask Display:
      | disp('Sloshing 1D \n mass-spring \n model(6x6)')
      | port_label('input', 1, 'Xddot')
      | port_label('output', 1, 'W_body/.')
  zaxis5 : Subsystem  AncestorBlock=SDTlibV1/6 dof bodies/u_sloshing  mask(Sloshing 1D mass-spring model(6x6)){xi=slosh.cj, w1=slosh.kj, m1=slosh.mj6}
      mask prompts: xi "Damping ratio"; w1 "Frequency (rd/s)"; m1 "Sloshing mass attached to the spring  (kg)"
      mask help:
      | Simplified dynamic model of lateral sloshing with a spring-mass model located at point P (connection point with the hub):
      | 6x6 transfer between acceleretion twist at P and wrench applied by the spring-mass system at P. The model is expressed in the (inherit) body frame.
      |
      | v: the direction vector of the spring-mass system.
      | Each parameter (except v) can be an uncertain parameter declared with "ureal"
      mask init:
      | % pass=ra2DCMi(v)
      mask Help: web('Docsloshing.html')
      mask DialogControl ParameterGroupVar Prompt: Main parameters
      mask DialogControl damping Prompt: Damping ratio
      mask DialogControl mode1 Prompt: Flexible mode:
      mask Display:
      | disp('Sloshing 1D \n mass-spring \n model(6x6)')
      | port_label('input', 1, 'Xddot')
      | port_label('output', 1, 'W_body/.')
  zaxis6 : Subsystem  AncestorBlock=SDTlibV1/6 dof bodies/u_sloshing  mask(Sloshing 1D mass-spring model(6x6)){xi=slosh.cj, w1=slosh.kj, m1=slosh.mj}
      mask prompts: xi "Damping ratio"; w1 "Frequency (rd/s)"; m1 "Sloshing mass attached to the spring  (kg)"
      mask help:
      | Simplified dynamic model of lateral sloshing with a spring-mass model located at point P (connection point with the hub):
      | 6x6 transfer between acceleretion twist at P and wrench applied by the spring-mass system at P. The model is expressed in the (inherit) body frame.
      |
      | v: the direction vector of the spring-mass system.
      | Each parameter (except v) can be an uncertain parameter declared with "ureal"
      mask init:
      | % pass=ra2DCMi(v)
      mask Help: web('Docsloshing.html')
      mask DialogControl ParameterGroupVar Prompt: Main parameters
      mask DialogControl damping Prompt: Damping ratio
      mask DialogControl mode1 Prompt: Flexible mode:
      mask Display:
      | disp('Sloshing 1D \n mass-spring \n model(6x6)')
      | port_label('input', 1, 'Xddot')
      | port_label('output', 1, 'W_body/.')
  Out2 : Outport
  wires:
  massless connection body1/1(W_body/.,P1) -> Out2/1
  In2/1 -> massless connection body1/1(Xddot,P1)
  massless connection body1/2(Xddot,P2) -> zaxis6/1(Xddot)
  zaxis6/1(W_body/.) -> massless connection body1/2(W_./body,P2)
  massless connection body1/3(Xddot,P3) -> zaxis1/1(Xddot)
  zaxis1/1(W_body/.) -> massless connection body1/3(W_./body,P3)
  zaxis4/1(W_body/.) -> massless connection body1/4(W_./body,P4)
  zaxis3/1(W_body/.) -> massless connection body1/5(W_./body,P5)
  zaxis2/1(W_body/.) -> massless connection body1/6(W_./body,P6)
  zaxis5/1(W_body/.) -> massless connection body1/7(W_./body,P7)
  massless connection body1/4(Xddot,P4) -> zaxis4/1(Xddot)
  massless connection body1/5(Xddot,P5) -> zaxis3/1(Xddot)
  massless connection body1/6(Xddot,P6) -> zaxis2/1(Xddot)
  massless connection body1/7(Xddot,P7) -> zaxis5/1(Xddot)

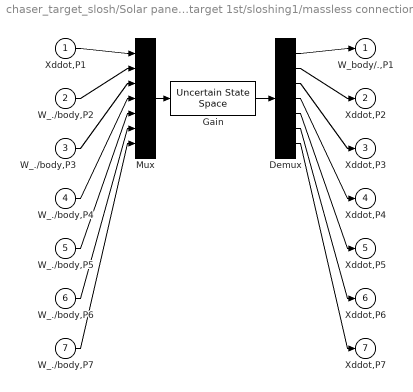
== system chaser_target_slosh/Solar panels target 1st/sloshing1/massless connection body1 ==
  Xddot,P1 : Inport  PortDimensions=6
  W_./body,P2 : Inport  Port=2  PortDimensions=6
  W_./body,P3 : Inport  Port=3  PortDimensions=6
  W_./body,P4 : Inport  Port=4  PortDimensions=6
  W_./body,P5 : Inport  Port=5  PortDimensions=6
  W_./body,P6 : Inport  Port=6  PortDimensions=6
  W_./body,P7 : Inport  Port=7  PortDimensions=6
  Demux : Demux  Outputs=[6 6 6 6 6 6 6]
  Gain : RCTblocks/Uncertain State Space  Tag=USS  USystem=uss(KIN)  UValue=[]  X0=[]  uX0=[]
  Mux : Mux  Inputs=[6 6 6 6 6 6 6]
  W_body/.,P1 : Outport
  Xddot,P2 : Outport  Port=2
  Xddot,P3 : Outport  Port=3
  Xddot,P4 : Outport  Port=4
  Xddot,P5 : Outport  Port=5
  Xddot,P6 : Outport  Port=6
  Xddot,P7 : Outport  Port=7
  wires:
  Mux/1 -> Gain/1
  Gain/1 -> Demux/1
  Xddot,P1/1 -> Mux/1
  Demux/1 -> W_body/.,P1/1
  W_./body,P2/1 -> Mux/2
  Demux/2 -> Xddot,P2/1
  W_./body,P3/1 -> Mux/3
  Demux/3 -> Xddot,P3/1
  W_./body,P4/1 -> Mux/4
  Demux/4 -> Xddot,P4/1
  W_./body,P5/1 -> Mux/5
  Demux/5 -> Xddot,P5/1
  W_./body,P6/1 -> Mux/6
  Demux/6 -> Xddot,P6/1
  W_./body,P7/1 -> Mux/7
  Demux/7 -> Xddot,P7/1

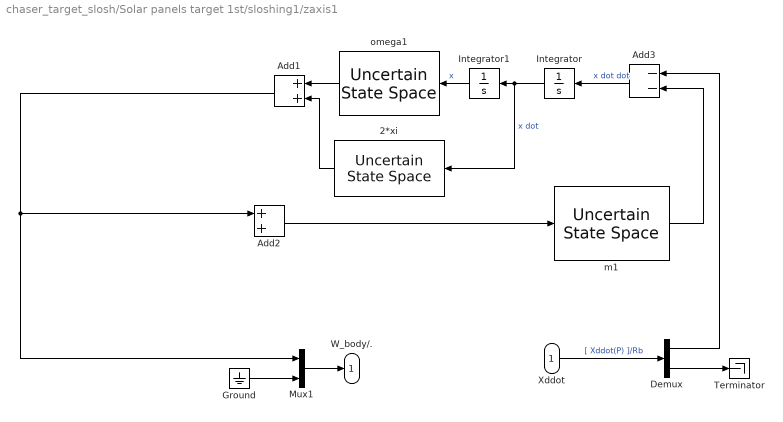
== system chaser_target_slosh/Solar panels target 1st/sloshing1/zaxis1 ==
  Xddot : Inport  PortDimensions=6
  2*xi : RCTblocks/Uncertain State Space  Tag=USS  USystem=uss(xi)*eye(3)  UValue=[]  X0=[]  uX0=[]
  Add1 : Sum
  Add2 : Sum
  Add3 : Sum  Inputs=--
  Demux : Demux  Outputs=[3 3]
  Ground : Ground
  Integrator : Integrator  InitialCondition=[0;0;0]
  Integrator1 : Integrator  InitialCondition=[0;0;0]
  Mux1 : Mux  Inputs=[3 3]
  Terminator : Terminator
  m1 : RCTblocks/Uncertain State Space  Tag=USS  USystem=1/uss(m1)*eye(3)  UValue=[]  X0=[]  uX0=[]
  "omega1 " : RCTblocks/Uncertain State Space  Tag=USS  USystem=uss(w1)*eye(3)  UValue=[]  X0=[]  uX0=[]
  W_body/. : Outport  PortDimensions=6  VectorParamsAs1DForOutWhenUnconnected=off
  wires:
  "omega1 "/1 -> Add1/1
  Integrator/1 -> 2*xi/1, Integrator1/1  "x dot"
  Integrator1/1 -> "omega1 "/1  "x"
  2*xi/1 -> Add1/2
  Mux1/1 -> W_body/./1
  Ground/1 -> Mux1/2
  Xddot/1 -> Demux/1  "[ Xddot(P) ]/Rb"
  Demux/2 -> Terminator/1
  Add3/1 -> Integrator/1  "x dot dot"
  Add1/1 -> Add2/1, Mux1/1
  Demux/1 -> Add3/1
  m1/1 -> Add3/2
  Add2/1 -> m1/1

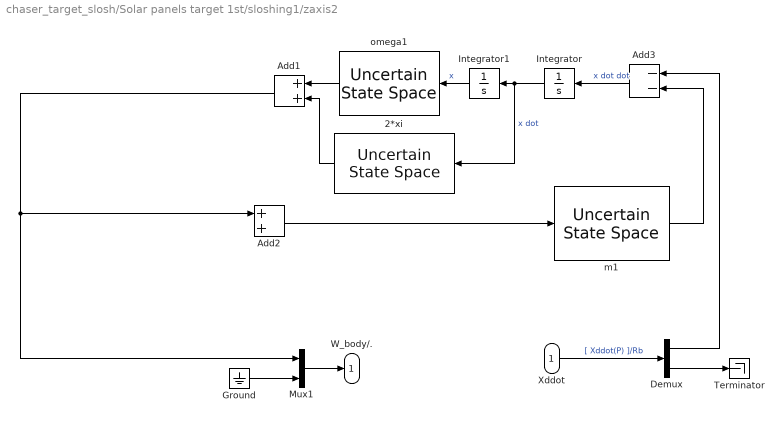
== system chaser_target_slosh/Solar panels target 1st/sloshing1/zaxis2 ==
  Xddot : Inport  PortDimensions=6
  2*xi : RCTblocks/Uncertain State Space  Tag=USS  USystem=uss(xi)*eye(3)  UValue=[]  X0=[]  uX0=[]
  Add1 : Sum
  Add2 : Sum
  Add3 : Sum  Inputs=--
  Demux : Demux  Outputs=[3 3]
  Ground : Ground
  Integrator : Integrator  InitialCondition=[0;0;0]
  Integrator1 : Integrator  InitialCondition=[0;0;0]
  Mux1 : Mux  Inputs=[3 3]
  Terminator : Terminator
  m1 : RCTblocks/Uncertain State Space  Tag=USS  USystem=1/uss(m1)*eye(3)  UValue=[]  X0=[]  uX0=[]
  "omega1 " : RCTblocks/Uncertain State Space  Tag=USS  USystem=uss(w1)*eye(3)  UValue=[]  X0=[]  uX0=[]
  W_body/. : Outport  PortDimensions=6  VectorParamsAs1DForOutWhenUnconnected=off
  wires:
  "omega1 "/1 -> Add1/1
  Integrator/1 -> 2*xi/1, Integrator1/1  "x dot"
  Integrator1/1 -> "omega1 "/1  "x"
  2*xi/1 -> Add1/2
  Mux1/1 -> W_body/./1
  Ground/1 -> Mux1/2
  Xddot/1 -> Demux/1  "[ Xddot(P) ]/Rb"
  Demux/2 -> Terminator/1
  Add3/1 -> Integrator/1  "x dot dot"
  Add1/1 -> Add2/1, Mux1/1
  Demux/1 -> Add3/1
  m1/1 -> Add3/2
  Add2/1 -> m1/1

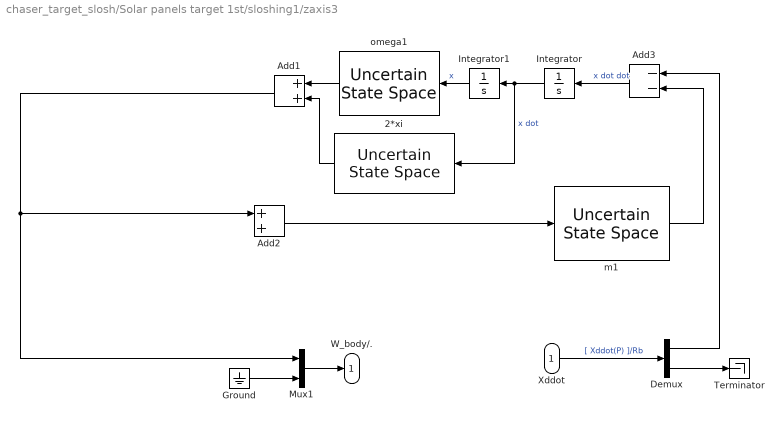
== system chaser_target_slosh/Solar panels target 1st/sloshing1/zaxis3 ==
  Xddot : Inport  PortDimensions=6
  2*xi : RCTblocks/Uncertain State Space  Tag=USS  USystem=uss(xi)*eye(3)  UValue=[]  X0=[]  uX0=[]
  Add1 : Sum
  Add2 : Sum
  Add3 : Sum  Inputs=--
  Demux : Demux  Outputs=[3 3]
  Ground : Ground
  Integrator : Integrator  InitialCondition=[0;0;0]
  Integrator1 : Integrator  InitialCondition=[0;0;0]
  Mux1 : Mux  Inputs=[3 3]
  Terminator : Terminator
  m1 : RCTblocks/Uncertain State Space  Tag=USS  USystem=1/uss(m1)*eye(3)  UValue=[]  X0=[]  uX0=[]
  "omega1 " : RCTblocks/Uncertain State Space  Tag=USS  USystem=uss(w1)*eye(3)  UValue=[]  X0=[]  uX0=[]
  W_body/. : Outport  PortDimensions=6  VectorParamsAs1DForOutWhenUnconnected=off
  wires:
  "omega1 "/1 -> Add1/1
  Integrator/1 -> 2*xi/1, Integrator1/1  "x dot"
  Integrator1/1 -> "omega1 "/1  "x"
  2*xi/1 -> Add1/2
  Mux1/1 -> W_body/./1
  Ground/1 -> Mux1/2
  Xddot/1 -> Demux/1  "[ Xddot(P) ]/Rb"
  Demux/2 -> Terminator/1
  Add3/1 -> Integrator/1  "x dot dot"
  Add1/1 -> Add2/1, Mux1/1
  Demux/1 -> Add3/1
  m1/1 -> Add3/2
  Add2/1 -> m1/1

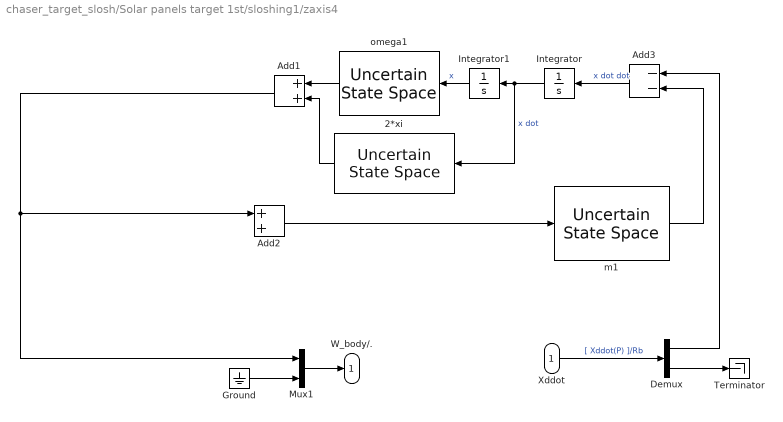
== system chaser_target_slosh/Solar panels target 1st/sloshing1/zaxis4 ==
  Xddot : Inport  PortDimensions=6
  2*xi : RCTblocks/Uncertain State Space  Tag=USS  USystem=uss(xi)*eye(3)  UValue=[]  X0=[]  uX0=[]
  Add1 : Sum
  Add2 : Sum
  Add3 : Sum  Inputs=--
  Demux : Demux  Outputs=[3 3]
  Ground : Ground
  Integrator : Integrator  InitialCondition=[0;0;0]
  Integrator1 : Integrator  InitialCondition=[0;0;0]
  Mux1 : Mux  Inputs=[3 3]
  Terminator : Terminator
  m1 : RCTblocks/Uncertain State Space  Tag=USS  USystem=1/uss(m1)*eye(3)  UValue=[]  X0=[]  uX0=[]
  "omega1 " : RCTblocks/Uncertain State Space  Tag=USS  USystem=uss(w1)*eye(3)  UValue=[]  X0=[]  uX0=[]
  W_body/. : Outport  PortDimensions=6  VectorParamsAs1DForOutWhenUnconnected=off
  wires:
  "omega1 "/1 -> Add1/1
  Integrator/1 -> 2*xi/1, Integrator1/1  "x dot"
  Integrator1/1 -> "omega1 "/1  "x"
  2*xi/1 -> Add1/2
  Mux1/1 -> W_body/./1
  Ground/1 -> Mux1/2
  Xddot/1 -> Demux/1  "[ Xddot(P) ]/Rb"
  Demux/2 -> Terminator/1
  Add3/1 -> Integrator/1  "x dot dot"
  Add1/1 -> Add2/1, Mux1/1
  Demux/1 -> Add3/1
  m1/1 -> Add3/2
  Add2/1 -> m1/1

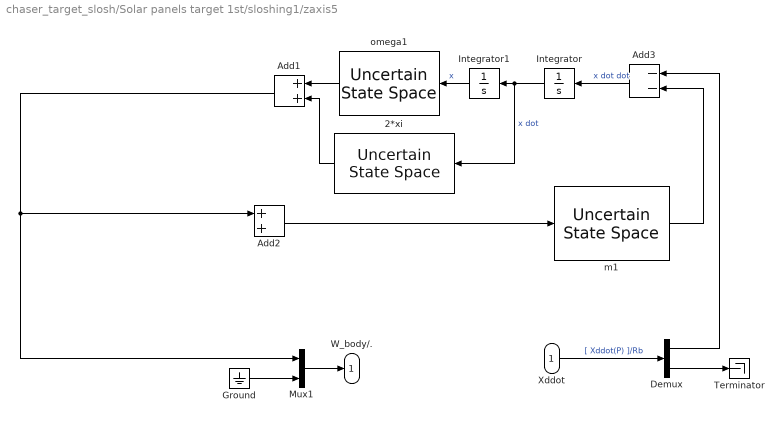
== system chaser_target_slosh/Solar panels target 1st/sloshing1/zaxis5 ==
  Xddot : Inport  PortDimensions=6
  2*xi : RCTblocks/Uncertain State Space  Tag=USS  USystem=uss(xi)*eye(3)  UValue=[]  X0=[]  uX0=[]
  Add1 : Sum
  Add2 : Sum
  Add3 : Sum  Inputs=--
  Demux : Demux  Outputs=[3 3]
  Ground : Ground
  Integrator : Integrator  InitialCondition=[0;0;0]
  Integrator1 : Integrator  InitialCondition=[0;0;0]
  Mux1 : Mux  Inputs=[3 3]
  Terminator : Terminator
  m1 : RCTblocks/Uncertain State Space  Tag=USS  USystem=1/uss(m1)*eye(3)  UValue=[]  X0=[]  uX0=[]
  "omega1 " : RCTblocks/Uncertain State Space  Tag=USS  USystem=uss(w1)*eye(3)  UValue=[]  X0=[]  uX0=[]
  W_body/. : Outport  PortDimensions=6  VectorParamsAs1DForOutWhenUnconnected=off
  wires:
  "omega1 "/1 -> Add1/1
  Integrator/1 -> 2*xi/1, Integrator1/1  "x dot"
  Integrator1/1 -> "omega1 "/1  "x"
  2*xi/1 -> Add1/2
  Mux1/1 -> W_body/./1
  Ground/1 -> Mux1/2
  Xddot/1 -> Demux/1  "[ Xddot(P) ]/Rb"
  Demux/2 -> Terminator/1
  Add3/1 -> Integrator/1  "x dot dot"
  Add1/1 -> Add2/1, Mux1/1
  Demux/1 -> Add3/1
  m1/1 -> Add3/2
  Add2/1 -> m1/1

== system chaser_target_slosh/Solar panels target 1st/sloshing1/zaxis6 ==
  Xddot : Inport  PortDimensions=6
  2*xi : RCTblocks/Uncertain State Space  Tag=USS  USystem=uss(xi)*eye(3)  UValue=[]  X0=[]  uX0=[]
  Add1 : Sum
  Add2 : Sum
  Add3 : Sum  Inputs=--
  Demux : Demux  Outputs=[3 3]
  Ground : Ground
  Integrator : Integrator  InitialCondition=[0;0;0]
  Integrator1 : Integrator  InitialCondition=[0;0;0]
  Mux1 : Mux  Inputs=[3 3]
  Terminator : Terminator
  m1 : RCTblocks/Uncertain State Space  Tag=USS  USystem=1/uss(m1)*eye(3)  UValue=[]  X0=[]  uX0=[]
  "omega1 " : RCTblocks/Uncertain State Space  Tag=USS  USystem=uss(w1)*eye(3)  UValue=[]  X0=[]  uX0=[]
  W_body/. : Outport  PortDimensions=6  VectorParamsAs1DForOutWhenUnconnected=off
  wires:
  "omega1 "/1 -> Add1/1
  Integrator/1 -> 2*xi/1, Integrator1/1  "x dot"
  Integrator1/1 -> "omega1 "/1  "x"
  2*xi/1 -> Add1/2
  Mux1/1 -> W_body/./1
  Ground/1 -> Mux1/2
  Xddot/1 -> Demux/1  "[ Xddot(P) ]/Rb"
  Demux/2 -> Terminator/1
  Add3/1 -> Integrator/1  "x dot dot"
  Add1/1 -> Add2/1, Mux1/1
  Demux/1 -> Add3/1
  m1/1 -> Add3/2
  Add2/1 -> m1/1

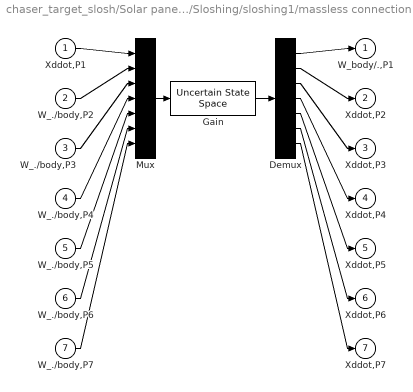
== system chaser_target_slosh/Solar panels//Sloshing/sloshing1/massless connection body1 ==
  Xddot,P1 : Inport  PortDimensions=6
  W_./body,P2 : Inport  Port=2  PortDimensions=6
  W_./body,P3 : Inport  Port=3  PortDimensions=6
  W_./body,P4 : Inport  Port=4  PortDimensions=6
  W_./body,P5 : Inport  Port=5  PortDimensions=6
  W_./body,P6 : Inport  Port=6  PortDimensions=6
  W_./body,P7 : Inport  Port=7  PortDimensions=6
  Demux : Demux  Outputs=[6 6 6 6 6 6 6]
  Gain : RCTblocks/Uncertain State Space  Tag=USS  USystem=uss(KIN)  UValue=[]  X0=[]  uX0=[]
  Mux : Mux  Inputs=[6 6 6 6 6 6 6]
  W_body/.,P1 : Outport
  Xddot,P2 : Outport  Port=2
  Xddot,P3 : Outport  Port=3
  Xddot,P4 : Outport  Port=4
  Xddot,P5 : Outport  Port=5
  Xddot,P6 : Outport  Port=6
  Xddot,P7 : Outport  Port=7
  wires:
  Mux/1 -> Gain/1
  Gain/1 -> Demux/1
  Xddot,P1/1 -> Mux/1
  Demux/1 -> W_body/.,P1/1
  W_./body,P2/1 -> Mux/2
  Demux/2 -> Xddot,P2/1
  W_./body,P3/1 -> Mux/3
  Demux/3 -> Xddot,P3/1
  W_./body,P4/1 -> Mux/4
  Demux/4 -> Xddot,P4/1
  W_./body,P5/1 -> Mux/5
  Demux/5 -> Xddot,P5/1
  W_./body,P6/1 -> Mux/6
  Demux/6 -> Xddot,P6/1
  W_./body,P7/1 -> Mux/7
  Demux/7 -> Xddot,P7/1

== system chaser_target_slosh/Solar panels//Sloshing/sloshing1/zaxis1 ==
  Xddot : Inport  PortDimensions=6
  2*xi : RCTblocks/Uncertain State Space  Tag=USS  USystem=uss(xi)*eye(3)  UValue=[]  X0=[]  uX0=[]
  Add1 : Sum
  Add2 : Sum
  Add3 : Sum  Inputs=--
  Demux : Demux  Outputs=[3 3]
  Ground : Ground
  Integrator : Integrator  InitialCondition=[0;0;0]
  Integrator1 : Integrator  InitialCondition=[0;0;0]
  Mux1 : Mux  Inputs=[3 3]
  Terminator : Terminator
  m1 : RCTblocks/Uncertain State Space  Tag=USS  USystem=1/uss(m1)*eye(3)  UValue=[]  X0=[]  uX0=[]
  "omega1 " : RCTblocks/Uncertain State Space  Tag=USS  USystem=uss(w1)*eye(3)  UValue=[]  X0=[]  uX0=[]
  W_body/. : Outport  PortDimensions=6  VectorParamsAs1DForOutWhenUnconnected=off
  wires:
  "omega1 "/1 -> Add1/1
  Integrator/1 -> 2*xi/1, Integrator1/1  "x dot"
  Integrator1/1 -> "omega1 "/1  "x"
  2*xi/1 -> Add1/2
  Mux1/1 -> W_body/./1
  Ground/1 -> Mux1/2
  Xddot/1 -> Demux/1  "[ Xddot(P) ]/Rb"
  Demux/2 -> Terminator/1
  Add3/1 -> Integrator/1  "x dot dot"
  Add1/1 -> Add2/1, Mux1/1
  Demux/1 -> Add3/1
  m1/1 -> Add3/2
  Add2/1 -> m1/1

== system chaser_target_slosh/Solar panels//Sloshing/sloshing1/zaxis2 ==
  Xddot : Inport  PortDimensions=6
  2*xi : RCTblocks/Uncertain State Space  Tag=USS  USystem=uss(xi)*eye(3)  UValue=[]  X0=[]  uX0=[]
  Add1 : Sum
  Add2 : Sum
  Add3 : Sum  Inputs=--
  Demux : Demux  Outputs=[3 3]
  Ground : Ground
  Integrator : Integrator  InitialCondition=[0;0;0]
  Integrator1 : Integrator  InitialCondition=[0;0;0]
  Mux1 : Mux  Inputs=[3 3]
  Terminator : Terminator
  m1 : RCTblocks/Uncertain State Space  Tag=USS  USystem=1/uss(m1)*eye(3)  UValue=[]  X0=[]  uX0=[]
  "omega1 " : RCTblocks/Uncertain State Space  Tag=USS  USystem=uss(w1)*eye(3)  UValue=[]  X0=[]  uX0=[]
  W_body/. : Outport  PortDimensions=6  VectorParamsAs1DForOutWhenUnconnected=off
  wires:
  "omega1 "/1 -> Add1/1
  Integrator/1 -> 2*xi/1, Integrator1/1  "x dot"
  Integrator1/1 -> "omega1 "/1  "x"
  2*xi/1 -> Add1/2
  Mux1/1 -> W_body/./1
  Ground/1 -> Mux1/2
  Xddot/1 -> Demux/1  "[ Xddot(P) ]/Rb"
  Demux/2 -> Terminator/1
  Add3/1 -> Integrator/1  "x dot dot"
  Add1/1 -> Add2/1, Mux1/1
  Demux/1 -> Add3/1
  m1/1 -> Add3/2
  Add2/1 -> m1/1

== system chaser_target_slosh/Solar panels//Sloshing/sloshing1/zaxis3 ==
  Xddot : Inport  PortDimensions=6
  2*xi : RCTblocks/Uncertain State Space  Tag=USS  USystem=uss(xi)*eye(3)  UValue=[]  X0=[]  uX0=[]
  Add1 : Sum
  Add2 : Sum
  Add3 : Sum  Inputs=--
  Demux : Demux  Outputs=[3 3]
  Ground : Ground
  Integrator : Integrator  InitialCondition=[0;0;0]
  Integrator1 : Integrator  InitialCondition=[0;0;0]
  Mux1 : Mux  Inputs=[3 3]
  Terminator : Terminator
  m1 : RCTblocks/Uncertain State Space  Tag=USS  USystem=1/uss(m1)*eye(3)  UValue=[]  X0=[]  uX0=[]
  "omega1 " : RCTblocks/Uncertain State Space  Tag=USS  USystem=uss(w1)*eye(3)  UValue=[]  X0=[]  uX0=[]
  W_body/. : Outport  PortDimensions=6  VectorParamsAs1DForOutWhenUnconnected=off
  wires:
  "omega1 "/1 -> Add1/1
  Integrator/1 -> 2*xi/1, Integrator1/1  "x dot"
  Integrator1/1 -> "omega1 "/1  "x"
  2*xi/1 -> Add1/2
  Mux1/1 -> W_body/./1
  Ground/1 -> Mux1/2
  Xddot/1 -> Demux/1  "[ Xddot(P) ]/Rb"
  Demux/2 -> Terminator/1
  Add3/1 -> Integrator/1  "x dot dot"
  Add1/1 -> Add2/1, Mux1/1
  Demux/1 -> Add3/1
  m1/1 -> Add3/2
  Add2/1 -> m1/1
